simulink model "CircShiftTest"  (R2023b)
settings: Solver=VariableStepAuto  StartTime=0.0  StopTime=1/260  RelTol=1e-3
settings Model: Creator=Koche  LastModifiedBy=Koche

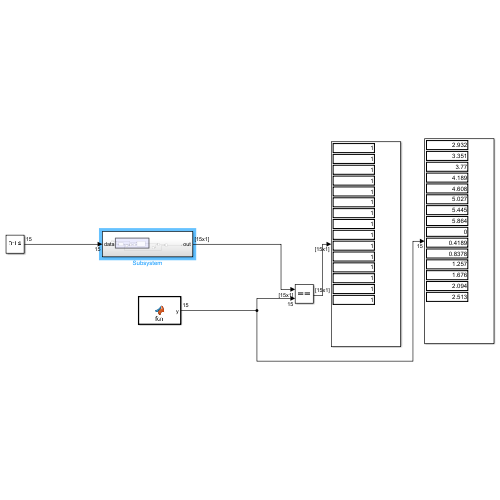
[thumbnail: Simulink's stored preview of the top-level diagram]
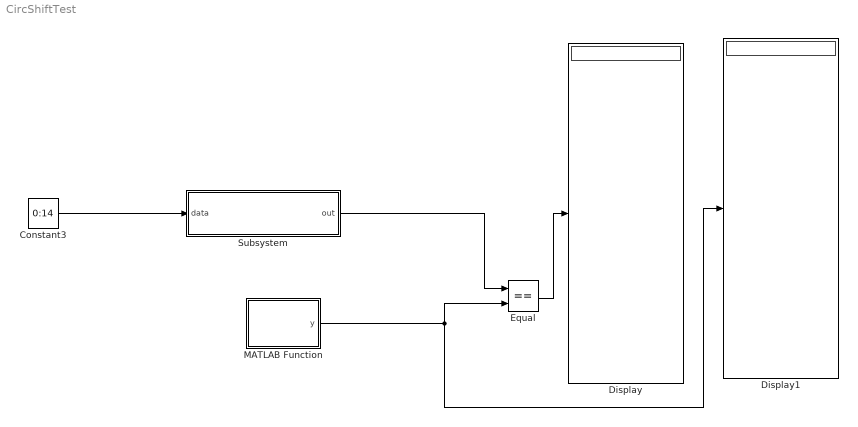
== system CircShiftTest ==
  Constant3 : Constant  Value=0:14  SampleTime=1/15
  Display : Display
  Display1 : Display
  Equal : RelationalOperator  Operator===  OutDataTypeStr=boolean  RndMeth=Simplest  InputSameDT=off
  MATLAB Function : MATLAB Function  TreatAsAtomicUnit=on
  Subsystem : Subsystem
  wires:
  Constant3/1 -> Subsystem/1(data)
  Subsystem/1(out) -> Equal/1
  MATLAB Function/1(y) -> Display1/1, Equal/2
  Equal/1 -> Display/1

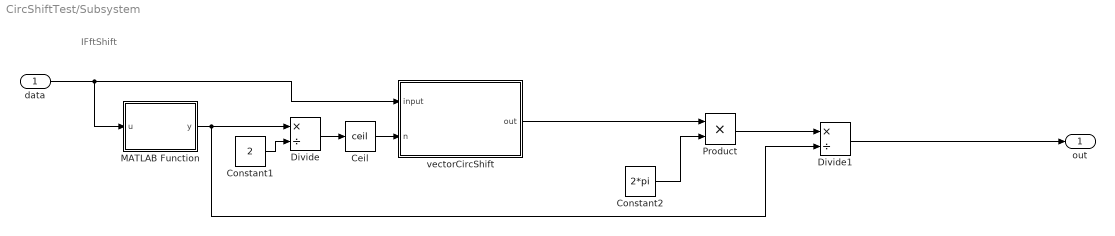
== system CircShiftTest/Subsystem ==
  note: IFftShift
  data : Inport
  " vectorCircShift" : Subsystem  mask{inputSize=15}
      mask prompts: inputSize "Input Size"
  Ceil : Rounding  Operator=ceil
  Constant1 : Constant  Value=2
  Constant2 : Constant  Value=2*pi
  Divide : Product  Inputs=*/  RndMeth=Zero  SaturateOnIntegerOverflow=on
  Divide1 : Product  Inputs=*/  RndMeth=Zero  SaturateOnIntegerOverflow=on
  MATLAB Function : MATLAB Function  TreatAsAtomicUnit=on
  Product : Product
  out : Outport
  wires:
  " vectorCircShift"/1(out) -> Product/1
  Constant2/1 -> Product/2
  Ceil/1 -> " vectorCircShift"/2(n)
  data/1 -> MATLAB Function/1(u), " vectorCircShift"/1(input)
  Constant1/1 -> Divide/2
  MATLAB Function/1(y) -> Divide1/2, Divide/1
  Divide/1 -> Ceil/1
  Product/1 -> Divide1/1
  Divide1/1 -> out/1

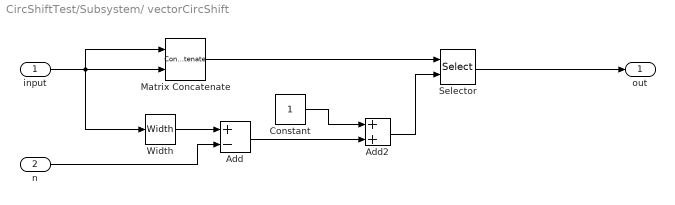
== system CircShiftTest/Subsystem/ vectorCircShift ==
  input : Inport
  n : Inport  Port=2
  Add : Sum  Inputs=+-
  Add2 : Sum
  Constant : Constant
  Matrix Concatenate : Concatenate  Mode=Multidimensional array
  Selector : Selector  NumberOfDimensions=2  InputPortWidth=30  IndexOptions=Starting index (port),Select all  Indices=[1 3],1  OutputSizes=inputSize,15
  Width : Width
  out : Outport
  wires:
  n/1 -> Add/2
  input/1 -> Width/1, Matrix Concatenate/2, Matrix Concatenate/1
  Matrix Concatenate/1 -> Selector/1
  Add/1 -> Add2/2
  Selector/1 -> out/1
  Width/1 -> Add/1
  Add2/1 -> Selector/2
  Constant/1 -> Add2/1

== matlab function CircShiftTest/Subsystem/MATLAB Function ==
  data: u input; y output
function y = fcn(u)
%#codegen

y = length(u);

== matlab function CircShiftTest/MATLAB Function ==
  data: y output
function y = fcn()
%#codegen

y  = 2*pi*ifftshift(((0:15-1)-0).')/15;
